simulink model "four_bots_CNN_DSM_compare"  (R2021a)
settings: Solver=ode5  StartTime=0.0  StopTime=30.0  FixedStep=0.001  RelTol=1e-3
(part 2 of 2)

== matlab function four_bots_CNN_DSM_compare/Multi agent System NN & SMC/Agent 4/Controller /Chebyshev neural network/Parameter Tuning ==
  data: phi_x input; xi input; W_dot output
function W_dot = parameter_tuning(phi_x, xi)

%% parameters that may alter
eta_1=0.1;

%% codes
W_dot = eta_1*phi_x*xi';

end

== matlab function four_bots_CNN_DSM_compare/Multi agent System NN & SMC/Agent 4/Controller /Chebyshev neural network/neural_initial ==
  data: weight output
function weight = neural_initialize()

% cheby_order   : order of chebyshev polynomials
% dimension     : dimension of the system

cheby_order=3;
dimension=3;

weight = zeros(1+2*cheby_order*dimension, dimension);

end

== matlab function four_bots_CNN_DSM_compare/Multi agent System NN & SMC/Agent 4/Controller /Control dot1 ==
  data: E_hat input; delta_v input; xi_i input; acc_d input; pi_dot output; acc_d_dot input; pi_i input
function pi_dot = control_dot(E_hat, delta_v, xi_i, acc_d, acc_d_dot , pi_i)

%% Basic parameters
dimension = 3;

%% Controller parameters
lambda = 2.5;
k = 2.5;
c = 10;

%% codes
pi_dot= -E_hat + acc_d_dot - (k + lambda) * (pi_i - acc_d) - k * lambda * delta_v - c * xi_i;

end

== matlab function four_bots_CNN_DSM_compare/Multi agent System NN & SMC/Agent 4/Controller /Dynamic Sliding Variable ==
  data: e_x input; xi output; e_v input; e_a input
function xi = sliding_variable(e_x, e_v, e_a)

%% parameters that may alter
k=2.5;
lambda=2.5;

%% codes
xi = e_a + (k + lambda)* e_v + lambda * k * e_x;

end

== matlab function four_bots_CNN_DSM_compare/Multi agent System NN & SMC/Agent 1 /Controller /Dynamic Sliding Variable ==
  data: e_x input; xi output; e_v input; e_a input
function xi = sliding_variable(e_x, e_v, e_a)

%% parameters that may alter
k=2.5;
lambda=2.5;

%% codes
xi = e_a + (k + lambda)* e_v + lambda * k * e_x;

end

== matlab function four_bots_CNN_DSM_compare/Multi agent System NN & SMC/Agent 1 /Controller /Control dot1 ==
  data: E_hat input; delta_v input; xi_i input; acc_d input; pi_dot output; acc_d_dot input; pi_i input
function pi_dot = control_dot(E_hat, delta_v, xi_i, acc_d, acc_d_dot , pi_i)

%% Basic parameters
dimension = 3;

%% Controller parameters
lambda = 2.5;
k = 2.5;
c = 10;

%% codes
pi_dot= -E_hat + acc_d_dot - (k + lambda) * (pi_i - acc_d) - k * lambda * delta_v - c * xi_i;

end

== matlab function four_bots_CNN_DSM_compare/Multi agent System NN & SMC/Agent 1 /Controller /Error Calculation1 ==
  data: current_states input; L input; delta_xi output; delta_vi output; reference input; e_x output; e_v output; e_a output; acc_d output; acc_d_dot output
function  [delta_xi, delta_vi, e_x, e_v, e_a, acc_d, acc_d_dot] = error_calculation(current_states, L, reference)

%% parameters that may change for alternative use
dimension = 3;
serial_num = 1;

num_agent = size(L,1);
%% current states
% Current states
pos = current_states(dimension*num_agent*0+1 : dimension*num_agent*1);
vel = current_states(dimension*num_agent*1+1 : dimension*num_agent*2);
acc = current_states(dimension*num_agent*2+1 : dimension*num_agent*3);

% Current reference
r_pos = reference(dimension*num_agent*0+1 : dimension*num_agent*1);
r_vel = reference(dimension*num_agent*1+1 : dimension*num_agent*2);
r_acc = reference(dimension*num_agent*2+1 : dimension*num_agent*3);
r_acc_dot = reference(dimension*num_agent*3+1 : dimension*num_agent*4);

%% Individual reference
acc_d = r_acc(dimension*(serial_num-1)+1 : dimension*serial_num);
acc_d_dot = r_acc_dot(dimension*(serial_num-1)+1 : dimension*serial_num);

%% Individual error
delta_x = pos - r_pos;
delta_v = vel - r_vel;

delta_xi = delta_x(dimension*(serial_num-1)+1 : dimension*serial_num);
delta_vi = delta_v(dimension*(serial_num-1)+1 : dimension*serial_num);

%% Local error
e_x = kron(L(serial_num, : ), eye(dimension) ) * (pos - r_pos);
e_v = kron(L(serial_num, : ), eye(dimension) ) * (vel - r_vel);
e_a = kron(L(serial_num, : ), eye(dimension) ) * (acc - r_acc);


end

== matlab function four_bots_CNN_DSM_compare/Multi agent System NN & SMC/Agent 4/Controller /Error Calculation1 ==
  data: current_states input; L input; delta_xi output; delta_vi output; reference input; e_x output; e_v output; e_a output; acc_d output; acc_d_dot output
function  [delta_xi, delta_vi, e_x, e_v, e_a, acc_d, acc_d_dot] = error_calculation(current_states, L, reference)

%% parameters that may change for alternative use
dimension = 3;
serial_num = 4;

num_agent = size(L,1);
%% current states
% Current states
pos = current_states(dimension*num_agent*0+1 : dimension*num_agent*1);
vel = current_states(dimension*num_agent*1+1 : dimension*num_agent*2);
acc = current_states(dimension*num_agent*2+1 : dimension*num_agent*3);

% Current reference
r_pos = reference(dimension*num_agent*0+1 : dimension*num_agent*1);
r_vel = reference(dimension*num_agent*1+1 : dimension*num_agent*2);
r_acc = reference(dimension*num_agent*2+1 : dimension*num_agent*3);
r_acc_dot = reference(dimension*num_agent*3+1 : dimension*num_agent*4);

%% Individual reference
acc_d = r_acc(dimension*(serial_num-1)+1 : dimension*serial_num);
acc_d_dot = r_acc_dot(dimension*(serial_num-1)+1 : dimension*serial_num);

%% Individual error
delta_x = pos - r_pos;
delta_v = vel - r_vel;

delta_xi = delta_x(dimension*(serial_num-1)+1 : dimension*serial_num);
delta_vi = delta_v(dimension*(serial_num-1)+1 : dimension*serial_num);

%% Local error
e_x = kron(L(serial_num, : ), eye(dimension) ) * (pos - r_pos);
e_v = kron(L(serial_num, : ), eye(dimension) ) * (vel - r_vel);
e_a = kron(L(serial_num, : ), eye(dimension) ) * (acc - r_acc);


end

== matlab function four_bots_CNN_DSM_compare/Multi agent System NN & SMC/Agent 4/Controller /Hysteresis/MATLAB Function1 ==
  data: u input; actual_control output; u_dot input; zeta input; zeta_dot output
function [actual_control, zeta_dot] = B_W_hysteresis(u, u_dot, zeta)

%% Hysteresis parameters
mu=1.5;
mu_bar=3;
chi_bar=1;
chi=0.5;
n=2;

actual_control=mu*u+mu_bar*zeta;

f=ones(3,1)-chi_bar*sign(u_dot).*abs(zeta).^(n-1).*zeta-chi*abs(zeta).^n;

zeta_dot=u_dot.*f;


end

== matlab function four_bots_CNN_DSM_compare/Multi agent System NN & SMC/Agent 4/Estimation error ==
  data: fx_dt input; error_norm output; fx_dtdot input; E input
function error_norm = estimation_error(fx_dt, fx_dtdot, E)

c=2.5;
lambda=2.5;

esti_error = fx_dtdot + (c + lambda) * fx_dt - E; 

error_norm = norm(esti_error); 

end

== matlab function four_bots_CNN_DSM_compare/Multi agent System NN & SMC/Agent 1 /Controller /Chebyshev neural network/MATLAB Function ==
  data: W input; W output
function W = smooth_projection(W)

%% smooth projection
Wmax=0.3;
Wmin=-0.3;
epsi=0.01;

for i=1:size(W,1)
   for j=1:size(W,2)
      if W(i,j)>Wmax
          W(i,j)=Wmax + epsi * (1-exp(-(W(i,j)-Wmax)/epsi));
      elseif W(i,j)<Wmin
          W(i,j)=Wmin - epsi * (1-exp((W(i,j)-Wmin)/epsi));
      else
          W(i,j)=W(i,j);
      end
   end
end

end

== matlab function four_bots_CNN_DSM_compare/Multi agent System NN & SMC/Agent 4/ODR model ==
  data: agent_x1 input; v_dot output; agent_x2 input; t input; control_input input; w_i output
function [v_dot, w_i] = physical_model( agent_x1 , agent_x2, t, control_input )

Mass=[4.5,5.2,4.8,5.5];
Radius=[0.20,0.24,0.22,0.26];
Inertia=[2.2,2.4,2.3,2.5]/10;
Beta=[11.4,11.6,11.8,12.0];

%% assign the parameter according to serial number
serial_num = 4; 
m=Mass(serial_num);
R=Radius(serial_num);
inertia=Inertia(serial_num);
beta=Beta(serial_num);

%% current states of the robot
x=agent_x1(1);
y=agent_x1(2);
theta=agent_x1(3);

%% the real model of robot
M=diag([1/m,1/m,1/inertia]);
T=[-sin(theta), -sin(pi/3-theta), sin(pi/3+theta);
    cos(theta), -cos(pi/3-theta), -cos(pi/3+theta);
    R,          R,                  R];

T_R = [-sin(theta), -sin(pi/3-theta), sin(pi/3+theta);
        cos(theta), -cos(pi/3-theta), -cos(pi/3+theta);
        1/R,          1/R,                  1/R];

real_fx = - beta * T * T_R^(-1) * M * agent_x2;
% real_fx = zeros(3,1);
bar_w_i = [0.3 * x * sin(t+pi/3*serial_num)+2; 0.2 * y * cos(2*t+pi/3*serial_num)+1.5; 0.1 * theta * sin(0.8*t+pi/3*serial_num)+1];

%% saturation is added here for convinience
% Vmax=6; % the maximum voltage of the motor
% 
% u1up=Vmax/(alpha*m)*(abs(sin(theta))+abs(sin(pi/3-theta))+abs(sin(pi/3+theta)));
% u1do=-Vmax/(alpha*m)*(abs(sin(theta))+abs(sin(pi/3-theta))+abs(sin(pi/3+theta)));
% u2up=Vmax/(alpha*m)*(abs(cos(theta))+abs(cos(pi/3-theta))+abs(cos(pi/3+theta)));
% u2do=-Vmax/(alpha*m)*(abs(cos(theta))+abs(cos(pi/3-theta))+abs(cos(pi/3+theta)));
% u3up=R/(alpha*inertia)*3*Vmax;
% u3do=-R/(alpha*inertia)*3*Vmax;
% 
% control_input(1) = max( min(control_input(1),u1up), u1do );
% control_input(2) = max( min(control_input(2),u2up), u2do );
% control_input(3) = max( min(control_input(3),u3up), u3do );


w_i = real_fx + bar_w_i; 

v_dot = control_input + w_i;


end

== matlab function four_bots_CNN_DSM_compare/Reference Generator/Acceleration reference ==
  data: t input; x2d_dot output
function x2d_dot = gene_ref_x2_dot(t)

%% generate position reference
radius_1=1;
radius_2=2;
w=0.1;

phase=0;
x1=[-radius_1*w^2*cos(w*t+pi/2*1+phase)-radius_2*w^2*cos(-w*t+pi/4) ; -radius_1*w^2*sin(w*t+pi/2*1+phase)+radius_2*w^2*sin(-w*t+pi/4) ; 0];
x2=[-radius_1*w^2*cos(w*t+pi/2*2+phase)-radius_2*w^2*cos(-w*t+pi/4) ; -radius_1*w^2*sin(w*t+pi/2*2+phase)+radius_2*w^2*sin(-w*t+pi/4) ; 0];
x3=[-radius_1*w^2*cos(w*t+pi/2*3+phase)-radius_2*w^2*cos(-w*t+pi/4) ; -radius_1*w^2*sin(w*t+pi/2*3+phase)+radius_2*w^2*sin(-w*t+pi/4) ; 0];
x4=[-radius_1*w^2*cos(w*t+pi/2*4+phase)-radius_2*w^2*cos(-w*t+pi/4) ; -radius_1*w^2*sin(w*t+pi/2*4+phase)+radius_2*w^2*sin(-w*t+pi/4) ; 0];

x2d_dot=[x1;x2;x3;x4];

== matlab function four_bots_CNN_DSM_compare/Reference Generator/Acceleration_dot Reference ==
  data: t input; x2ddot output
function x2ddot = gene_ref_x2ddot(t)

%% generate position reference
radius_1=1;
radius_2=2;
w=0.1;

phase=0;
x1=[radius_1*w^3*sin(w*t+pi/2*1+phase)-radius_2*w^3*sin(-w*t+pi/4) ; -radius_1*w^3*cos(w*t+pi/2*1+phase)-radius_2*w^3*cos(-w*t+pi/4) ; 0];
x2=[radius_1*w^3*sin(w*t+pi/2*2+phase)-radius_2*w^3*sin(-w*t+pi/4) ; -radius_1*w^3*cos(w*t+pi/2*2+phase)-radius_2*w^3*cos(-w*t+pi/4) ; 0];
x3=[radius_1*w^3*sin(w*t+pi/2*3+phase)-radius_2*w^3*sin(-w*t+pi/4) ; -radius_1*w^3*cos(w*t+pi/2*3+phase)-radius_2*w^3*cos(-w*t+pi/4) ; 0];
x4=[radius_1*w^3*sin(w*t+pi/2*4+phase)-radius_2*w^3*sin(-w*t+pi/4) ; -radius_1*w^3*cos(w*t+pi/2*4+phase)-radius_2*w^3*cos(-w*t+pi/4) ; 0];

x2ddot=[x1;x2;x3;x4];

== matlab function four_bots_CNN_DSM_compare/Reference Generator/Position Reference ==
  data: t input; x1d output
function x1d = gene_ref_x1(t)

%% generate position reference
radius_1=1;
radius_2=2;
w=0.1;

phase=0;

x1=[radius_1*cos(w*t+pi/2*1+phase)+radius_2*cos(-w*t+pi/4) ; radius_1*sin(w*t+pi/2*1+phase)+radius_2*sin(-w*t+pi/4) ; 1*pi/4];
x2=[radius_1*cos(w*t+pi/2*2+phase)+radius_2*cos(-w*t+pi/4) ; radius_1*sin(w*t+pi/2*2+phase)+radius_2*sin(-w*t+pi/4) ; 2*pi/4];
x3=[radius_1*cos(w*t+pi/2*3+phase)+radius_2*cos(-w*t+pi/4) ; radius_1*sin(w*t+pi/2*3+phase)+radius_2*sin(-w*t+pi/4) ; 3*pi/4];
x4=[radius_1*cos(w*t+pi/2*4+phase)+radius_2*cos(-w*t+pi/4) ; radius_1*sin(w*t+pi/2*4+phase)+radius_2*sin(-w*t+pi/4) ; 4*pi/4];

x1d=[x1;x2;x3;x4];

== matlab function four_bots_CNN_DSM_compare/Reference Generator/Speed Reference ==
  data: t input; x2d output
function x2d = gene_ref_x2(t)

%% generate position reference
radius_1=1;
radius_2=2;
w=0.1;

phase=0;

x1=[-radius_1*w*sin(w*t+pi/2*1+phase)+radius_2*w*sin(-w*t+pi/4) ; radius_1*w*cos(w*t+pi/2*1+phase)-radius_2*w*cos(-w*t+pi/4) ; 0];
x2=[-radius_1*w*sin(w*t+pi/2*2+phase)+radius_2*w*sin(-w*t+pi/4) ; radius_1*w*cos(w*t+pi/2*2+phase)-radius_2*w*cos(-w*t+pi/4) ; 0];
x3=[-radius_1*w*sin(w*t+pi/2*3+phase)+radius_2*w*sin(-w*t+pi/4) ; radius_1*w*cos(w*t+pi/2*3+phase)-radius_2*w*cos(-w*t+pi/4) ; 0];
x4=[-radius_1*w*sin(w*t+pi/2*4+phase)+radius_2*w*sin(-w*t+pi/4) ; radius_1*w*cos(w*t+pi/2*4+phase)-radius_2*w*cos(-w*t+pi/4) ; 0];

x2d=[x1;x2;x3;x4];

== matlab function four_bots_CNN_DSM_compare/Multi agent System NN & SMC/Agent 1 /Controller /Chebyshev neural network/Estimation ==
  data: phi_x input; W input; E output
function E = estimation(phi_x, W)
%% estimation
E=W'*phi_x;

end

== matlab function four_bots_CNN_DSM_compare/Multi agent System NN & SMC/Agent 1 /Controller /Hysteresis/MATLAB Function1 ==
  data: u input; actual_control output; u_dot input; zeta input; zeta_dot output
function [actual_control, zeta_dot] = B_W_hysteresis(u, u_dot, zeta)

%% Hysteresis parameters
mu=1.5;
mu_bar=3;
chi_bar=1;
chi=0.5;
n=2;

actual_control=mu*u+mu_bar*zeta;

f=ones(3,1)-chi_bar*sign(u_dot).*abs(zeta).^(n-1).*zeta-chi*abs(zeta).^n;

zeta_dot=u_dot.*f;


end

== matlab function four_bots_CNN_DSM_compare/Multi agent System NN & SMC/Agent 2/Controller /Chebyshev neural network/Chebyshev Polynomials ==
  data: current_states input; phi_x output
function phi_x = Chebyshev_polynomials(current_states)

%% parameters that may alter
dimension=3;
cheby_order=3;

%% current states
x1=current_states(dimension*0+1:dimension*1);
x2=current_states(dimension*1+1:dimension*2);

%% initialization
phi_x=ones(1+2*dimension*cheby_order,1);

%% recursion procedure
now_x=[x1;x2];
for order = 1 : cheby_order
   if order == 1
      phi_x(2*dimension*(order-1)+2:2*dimension*order+1)=now_x;
   elseif order == 2
      phi_x(2*dimension*(order-1)+2:2*dimension*order+1)=2*now_x.*phi_x(2*dimension*(order-2)+2:2*dimension*(order-1)+1)-1;
   else
      phi_x(2*dimension*(order-1)+2:2*dimension*order+1)=2*now_x.*phi_x(2*dimension*(order-2)+2:2*dimension*(order-1)+1)-phi_x(2*dimension*(order-3)+2:2*dimension*(order-2)+1);
   end
end

end

== matlab function four_bots_CNN_DSM_compare/Multi agent System NN & SMC/Agent 2/Controller /Chebyshev neural network/Estimation ==
  data: phi_x input; W input; E output
function E = estimation(phi_x, W)
%% estimation
E=W'*phi_x;

end

== matlab function four_bots_CNN_DSM_compare/Multi agent System NN & SMC/Agent 2/Controller /Chebyshev neural network/MATLAB Function ==
  data: W input; W output
function W = smooth_projection(W)

%% smooth projection
Wmax=0.3;
Wmin=-0.3;
epsi=0.01;

for i=1:size(W,1)
   for j=1:size(W,2)
      if W(i,j)>Wmax
          W(i,j)=Wmax + epsi * (1-exp(-(W(i,j)-Wmax)/epsi));
      elseif W(i,j)<Wmin
          W(i,j)=Wmin - epsi * (1-exp((W(i,j)-Wmin)/epsi));
      else
          W(i,j)=W(i,j);
      end
   end
end

end

== matlab function four_bots_CNN_DSM_compare/Multi agent System NN & SMC/Agent 2/Controller /Chebyshev neural network/Parameter Tuning ==
  data: phi_x input; xi input; W_dot output
function W_dot = parameter_tuning(phi_x, xi)

%% parameters that may alter
eta_1=0.1;

%% codes
W_dot = eta_1*phi_x*xi';

end

== matlab function four_bots_CNN_DSM_compare/Multi agent System NN & SMC/Agent 2/Controller /Chebyshev neural network/neural_initial ==
  data: weight output
function weight = neural_initialize()

% cheby_order   : order of chebyshev polynomials
% dimension     : dimension of the system

cheby_order=3;
dimension=3;

weight = zeros(1+2*cheby_order*dimension, dimension);

end
